simulink model "w2project3_2019a"  (R2019a)
settings: Solver=VariableStepAuto  StartTime=0.0  StopTime=10.0  RelTol=1e-3
model workspace (MAT data in the model file):
  Ki = 40
  Kp = 800
  b = 50
  m = 1000
  u = 500
settings Model: Creator=rutvi  LastModifiedBy=rutvi
settings SolverCC: AlgebraicLoopSolver=LineSearch

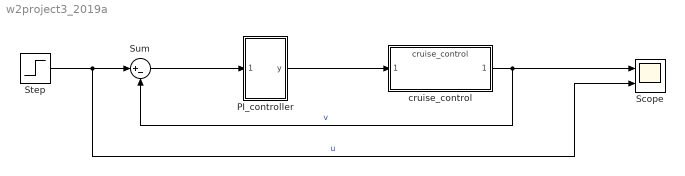
== system w2project3_2019a ==
  PI_controller : Subsystem
  Scope : Scope  NumInputPorts=2
  Step : Step  After=u  SampleTime=0
  Sum : Sum  Inputs=|+-
  cruise_control : ModelReference  ModelNameDialog=cruise_control  SimulationMode=Normal  ModelReferenceVersion=1.2
  wires:
  cruise_control/1 -> Scope/1, Sum/2  "v"
  Step/1 -> Sum/1, Scope/2  "u"
  Sum/1 -> PI_controller/1(error)
  PI_controller/1(y) -> cruise_control/1

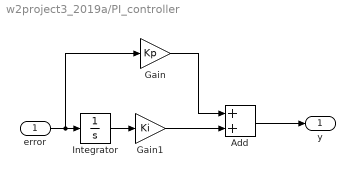
== system w2project3_2019a/PI_controller ==
  error : Inport
  Add : Sum
  Gain : Gain  Gain=Kp
  Gain1 : Gain  Gain=Ki
  Integrator : Integrator
  y : Outport
  wires:
  Add/1 -> y/1
  Integrator/1 -> Gain1/1
  error/1 -> Gain/1, Integrator/1
  Gain1/1 -> Add/2
  Gain/1 -> Add/1
